simulink library "xps_library"  (R2021a)
settings: Solver=VariableStepAuto  StartTime=0.0  StopTime=10.0  RelTol=1e-3
undefined symbols (not defined in the file): ip_name, lib_path
libraries: xbsIndex_r4 x2612, casper_library_flow_control x68, simulink x52, $bdroot x9, casper_library_misc x9
(part 6 of 33)

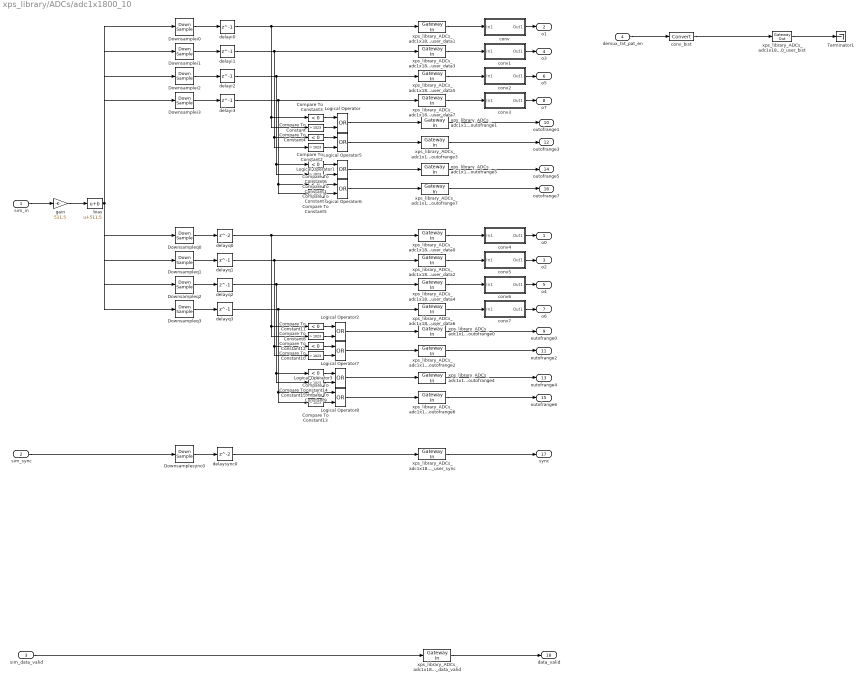
== system xps_library/ADCs/adc1x1800_10 ==
  sim_in : Inport  SampleTime=sample_period/8
  sim_sync : Inport  Port=2  SampleTime=sample_period/8
  sim_data_valid : Inport  Port=3  SampleTime=sample_period/4
  demux_tst_pat_en : Inport  Port=4  SampleTime=sample_period/8
  Compare To Constant{,1..2,5,8..10,13} (8 alike) : simulink/Logic and Bit Operations/Compare To Constant  relop=>  const=1023  OutDataTypeStr=boolean  ZeroCross=off
  Compare To Constant{3..4,6..7,11..12,14..15} (8 alike) : simulink/Logic and Bit Operations/Compare To Constant  relop=<  const=0  OutDataTypeStr=boolean  ZeroCross=off
  Downsamplei0 : DownSample  N=8  phase=1  InputProcessing=Inherited (this choice will be removed - see release notes)
  Downsamplei1 : DownSample  N=8  phase=3  InputProcessing=Inherited (this choice will be removed - see release notes)
  Downsamplei2 : DownSample  N=8  phase=5  InputProcessing=Inherited (this choice will be removed - see release notes)
  Downsamplei3 : DownSample  N=8  phase=7  InputProcessing=Inherited (this choice will be removed - see release notes)
  Downsampleq0 : DownSample  N=8  InputProcessing=Inherited (this choice will be removed - see release notes)
  Downsampleq1 : DownSample  N=8  phase=2  InputProcessing=Inherited (this choice will be removed - see release notes)
  Downsampleq2 : DownSample  N=8  phase=4  InputProcessing=Inherited (this choice will be removed - see release notes)
  Downsampleq3 : DownSample  N=8  phase=6  InputProcessing=Inherited (this choice will be removed - see release notes)
  Downsamplesync0 : DownSample  N=8  InputProcessing=Inherited (this choice will be removed - see release notes)
  Logical Operator{,1..3,5..8} (8 alike) : Logic  Operator=OR  AllPortsSameDT=off  OutDataTypeStr=boolean
  Terminator1 : Terminator
  bias : Bias  Bias=511.5  SaturateOnIntegerOverflow=on
  conv : Subsystem
  conv1 : Subsystem
  conv2 : Subsystem
  conv3 : Subsystem
  conv4 : Subsystem
  conv5 : Subsystem
  conv6 : Subsystem
  conv7 : Subsystem
  conv_bist : xbsIndex_r4/Convert  gui_display_data_type=Fixed-point  arith_type=Boolean  n_bits=8  bin_pt=0  float_type=Single  exp_bits=8  fraction_bits=24  quantization=Truncate  overflow=Wrap  en=off  latency=0  pipeline=off  dbl_ovrd=off  block_type=convert
      settings: xl_area=[0, 0, 0, 0, 0, 0, 0]
  delayi{0..3} (4 alike) : Delay  DelayLength=1
  delayq0 : Delay
  delayq1 : Delay  DelayLength=1
  delayq2 : Delay  DelayLength=1
  delayq3 : Delay  DelayLength=1
  delaysync0 : Delay
  gain : Gain  Gain=511.5  SaturateOnIntegerOverflow=on  OutDataTypeStr=Inherit: Same as input  ParamDataTypeStr=Inherit: Same as input
  xps_library_ADCs_adc1x1800_10_user_bist : xbsIndex_r4/Gateway Out  inherit_from_input=off  hdl_port=on  rows=1  columns=1  UseAsDAC=off  DACChannel='1'  interface=None  automatic_assignment=on  address_offset=hex2dec('00')  intf_name=''  intf_description=''  timing_constraint=None  locs_specified=off  LOCs={}  io_standard={}  block_type=gatewayout
      settings: infoedit="Gateway out block.  Converts Xilinx fixed point inputs into ouputs of type Simulink integer, double, or fixed point.<br><br>Hardware notes:  In hardware these blocks become top level output ports or are discarded, depending on how they are configured."  block_version=11.4
  xps_library_ADCs_adc1x1800_10_user_data{0..7} (8 alike) : xbsIndex_r4/Gateway In  gui_display_data_type=Fixed-point  arith_type=Unsigned  n_bits=10  bin_pt=0  preci_type=Single  exp_width=8  frac_width=24  rows=1  columns=1  quantization="Round  (unbiased: +/- Inf)"  overflow=Saturate  period=sample_period  UseAsADC=off  ADCChannel='1'  interface=None  automatic_assignment=on  address_offset=hex2dec('00')  intf_name=''  intf_description=''  default_value=0  timing_constraint=None  locs_specified=off  LOCs={}  io_standard={}  inherit_from_input=off  hdl_port=on  dbl_ovrd=off  block_type=gatewayin
      settings: infoedit="Gateway in block.  Converts inputs of type Simulink integer, double and fixed point to  Xilinx fixed point type.<br><br>Hardware notes:  In hardware these blocks become top level input ports."  xl_area=[0 0 0 0 8 0 0]  block_version=8.2.02
  xps_library_ADCs_adc1x1800_10_user_data_valid : xbsIndex_r4/Gateway In  gui_display_data_type=Fixed-point  arith_type=Boolean  n_bits=8  bin_pt=0  preci_type=Single  exp_width=8  frac_width=24  rows=1  columns=1  quantization="Round  (unbiased: +/- Inf)"  overflow=Saturate  period=sample_period  UseAsADC=off  ADCChannel='1'  interface=None  automatic_assignment=on  address_offset=hex2dec('00')  intf_name=''  intf_description=''  default_value=0  timing_constraint=None  locs_specified=off  LOCs={}  io_standard={}  inherit_from_input=off  hdl_port=on  dbl_ovrd=off  block_type=gatewayin
      settings: infoedit="Gateway in block.  Converts inputs of type Simulink integer, double and fixed point to  Xilinx fixed point type.<P><P>Hardware notes:  In hardware these blocks become top level input ports."  xl_area=[0 0 0 0 8 0 0]  block_version=8.2.02
  xps_library_ADCs_adc1x1800_10_user_outofrange{0..7} (8 alike) : xbsIndex_r4/Gateway In  gui_display_data_type=Fixed-point  arith_type=Boolean  n_bits=8  bin_pt=0  preci_type=Single  exp_width=8  frac_width=24  rows=1  columns=1  quantization="Round  (unbiased: +/- Inf)"  overflow=Saturate  period=sample_period  UseAsADC=off  ADCChannel='1'  interface=None  automatic_assignment=on  address_offset=hex2dec('00')  intf_name=''  intf_description=''  default_value=0  timing_constraint=None  locs_specified=off  LOCs={}  io_standard={}  inherit_from_input=off  hdl_port=on  dbl_ovrd=off  block_type=gatewayin
      settings: infoedit="Gateway in block.  Converts inputs of type Simulink integer, double and fixed point to  Xilinx fixed point type.<P><P>Hardware notes:  In hardware these blocks become top level input ports."  xl_area=[0 0 0 0 8 0 0]  block_version=8.2.02
  xps_library_ADCs_adc1x1800_10_user_sync : xbsIndex_r4/Gateway In  gui_display_data_type=Fixed-point  arith_type=Boolean  n_bits=8  bin_pt=0  preci_type=Single  exp_width=8  frac_width=24  rows=1  columns=1  quantization="Round  (unbiased: +/- Inf)"  overflow=Saturate  period=sample_period  UseAsADC=off  ADCChannel='1'  interface=None  automatic_assignment=on  address_offset=hex2dec('00')  intf_name=''  intf_description=''  default_value=0  timing_constraint=None  locs_specified=off  LOCs={}  io_standard={}  inherit_from_input=off  hdl_port=on  dbl_ovrd=off  block_type=gatewayin
      settings: infoedit="Gateway in block.  Converts inputs of type Simulink integer, double and fixed point to  Xilinx fixed point type.<P><P>Hardware notes:  In hardware these blocks become top level input ports."  xl_area=[0 0 0 0 8 0 0]  block_version=8.2.02
  o0 : Outport
  o1 : Outport  Port=2
  o2 : Outport  Port=3
  o3 : Outport  Port=4
  o4 : Outport  Port=5
  o5 : Outport  Port=6
  o6 : Outport  Port=7
  o7 : Outport  Port=8
  outofrange0 : Outport  Port=9
  outofrange1 : Outport  Port=10
  outofrange2 : Outport  Port=11
  outofrange3 : Outport  Port=12
  outofrange4 : Outport  Port=13
  outofrange5 : Outport  Port=14
  outofrange6 : Outport  Port=15
  outofrange7 : Outport  Port=16
  sync : Outport  Port=17
  data_valid : Outport  Port=18
  wires:
  delayq3/1 -> xps_library_ADCs_adc1x1800_10_user_data6/1, Compare To Constant15/1, Compare To Constant13/1
  delayq2/1 -> xps_library_ADCs_adc1x1800_10_user_data4/1, Compare To Constant14/1, Compare To Constant9/1
  delayq1/1 -> xps_library_ADCs_adc1x1800_10_user_data2/1, Compare To Constant12/1, Compare To Constant10/1
  delayi3/1 -> xps_library_ADCs_adc1x1800_10_user_data7/1, Compare To Constant7/1, Compare To Constant5/1
  delayi2/1 -> xps_library_ADCs_adc1x1800_10_user_data5/1, Compare To Constant6/1, Compare To Constant1/1
  delayi1/1 -> xps_library_ADCs_adc1x1800_10_user_data3/1, Compare To Constant2/1, Compare To Constant4/1
  Downsamplei0/1 -> delayi0/1
  xps_library_ADCs_adc1x1800_10_user_data6/1 -> conv7/1(In1)
  xps_library_ADCs_adc1x1800_10_user_data4/1 -> conv6/1(In1)
  xps_library_ADCs_adc1x1800_10_user_data2/1 -> conv5/1(In1)
  xps_library_ADCs_adc1x1800_10_user_data0/1 -> conv4/1(In1)
  xps_library_ADCs_adc1x1800_10_user_sync/1 -> sync/1
  xps_library_ADCs_adc1x1800_10_user_outofrange1/1 -> outofrange1/1
  xps_library_ADCs_adc1x1800_10_user_data7/1 -> conv3/1(In1)
  xps_library_ADCs_adc1x1800_10_user_data5/1 -> conv2/1(In1)
  xps_library_ADCs_adc1x1800_10_user_data3/1 -> conv1/1(In1)
  Downsampleq3/1 -> delayq3/1
  Downsampleq2/1 -> delayq2/1
  Downsampleq1/1 -> delayq1/1
  Downsamplei3/1 -> delayi3/1
  Downsamplei2/1 -> delayi2/1
  Downsamplei1/1 -> delayi1/1
  delayi0/1 -> xps_library_ADCs_adc1x1800_10_user_data1/1, Compare To Constant/1, Compare To Constant3/1
  Downsampleq0/1 -> delayq0/1
  delayq0/1 -> xps_library_ADCs_adc1x1800_10_user_data0/1, Compare To Constant11/1, Compare To Constant8/1
  Compare To Constant3/1 -> Logical Operator/1
  Compare To Constant/1 -> Logical Operator/2
  Compare To Constant4/1 -> Logical Operator5/1
  Compare To Constant2/1 -> Logical Operator5/2
  Logical Operator/1 -> xps_library_ADCs_adc1x1800_10_user_outofrange1/1
  Compare To Constant6/1 -> Logical Operator1/1
  Compare To Constant1/1 -> Logical Operator1/2
  Compare To Constant7/1 -> Logical Operator6/1
  Compare To Constant5/1 -> Logical Operator6/2
  Compare To Constant11/1 -> Logical Operator2/1
  Compare To Constant8/1 -> Logical Operator2/2
  Compare To Constant12/1 -> Logical Operator7/1
  Compare To Constant10/1 -> Logical Operator7/2
  Compare To Constant14/1 -> Logical Operator3/1
  Compare To Constant9/1 -> Logical Operator3/2
  Compare To Constant15/1 -> Logical Operator8/1
  Compare To Constant13/1 -> Logical Operator8/2
  sim_sync/1 -> Downsamplesync0/1
  Downsamplesync0/1 -> delaysync0/1
  delaysync0/1 -> xps_library_ADCs_adc1x1800_10_user_sync/1
  xps_library_ADCs_adc1x1800_10_user_data1/1 -> conv/1(In1)
  sim_in/1 -> gain/1
  gain/1 -> bias/1
  bias/1 -> Downsamplei0/1, Downsamplei1/1, Downsamplei2/1, Downsamplei3/1, Downsampleq0/1, Downsampleq1/1, Downsampleq2/1, Downsampleq3/1
  xps_library_ADCs_adc1x1800_10_user_outofrange3/1 -> outofrange3/1
  Logical Operator5/1 -> xps_library_ADCs_adc1x1800_10_user_outofrange3/1
  xps_library_ADCs_adc1x1800_10_user_outofrange5/1 -> outofrange5/1
  Logical Operator1/1 -> xps_library_ADCs_adc1x1800_10_user_outofrange5/1
  xps_library_ADCs_adc1x1800_10_user_outofrange7/1 -> outofrange7/1
  Logical Operator6/1 -> xps_library_ADCs_adc1x1800_10_user_outofrange7/1
  xps_library_ADCs_adc1x1800_10_user_outofrange0/1 -> outofrange0/1
  Logical Operator2/1 -> xps_library_ADCs_adc1x1800_10_user_outofrange0/1
  xps_library_ADCs_adc1x1800_10_user_outofrange2/1 -> outofrange2/1
  Logical Operator7/1 -> xps_library_ADCs_adc1x1800_10_user_outofrange2/1
  xps_library_ADCs_adc1x1800_10_user_outofrange4/1 -> outofrange4/1
  Logical Operator3/1 -> xps_library_ADCs_adc1x1800_10_user_outofrange4/1
  xps_library_ADCs_adc1x1800_10_user_outofrange6/1 -> outofrange6/1
  Logical Operator8/1 -> xps_library_ADCs_adc1x1800_10_user_outofrange6/1
  xps_library_ADCs_adc1x1800_10_user_data_valid/1 -> data_valid/1
  sim_data_valid/1 -> xps_library_ADCs_adc1x1800_10_user_data_valid/1
  demux_tst_pat_en/1 -> conv_bist/1
  xps_library_ADCs_adc1x1800_10_user_bist/1 -> Terminator1/1
  conv_bist/1 -> xps_library_ADCs_adc1x1800_10_user_bist/1
  conv/1(Out1) -> o1/1
  conv1/1(Out1) -> o3/1
  conv2/1(Out1) -> o5/1
  conv3/1(Out1) -> o7/1
  conv4/1(Out1) -> o0/1
  conv5/1(Out1) -> o2/1
  conv6/1(Out1) -> o4/1
  conv7/1(Out1) -> o6/1

== system xps_library/ADCs/adc2x14_400 ==
  conv : Subsystem
      mask help:
      | Converts an (12-bit) unsigned number to 2's complement.
      | This block should eventually be able to handle arbitrary
      | width inputs.
  conv1 : Subsystem
      mask help:
      | Converts an (12-bit) unsigned number to 2's complement.
      | This block should eventually be able to handle arbitrary
      | width inputs.
  conv2 : Subsystem
      mask help:
      | Converts an (12-bit) unsigned number to 2's complement.
      | This block should eventually be able to handle arbitrary
      | width inputs.
  conv3 : Subsystem
      mask help:
      | Converts an (12-bit) unsigned number to 2's complement.
      | This block should eventually be able to handle arbitrary
      | width inputs.
  xps_library_ADCs_adc2x14_400_user_data_i0 : xbsIndex_r4/Gateway In  gui_display_data_type=Fixed-point  arith_type=Unsigned  n_bits=14  bin_pt=0  preci_type=Single  exp_width=8  frac_width=24  rows=1  columns=1  quantization=Truncate  overflow=Wrap  period=1  UseAsADC=off  ADCChannel='1'  interface=None  automatic_assignment=on  address_offset=hex2dec('00')  intf_name=''  intf_description=''  default_value=0  timing_constraint=None  locs_specified=off  LOCs={}  io_standard={}  inherit_from_input=off  hdl_port=on  dbl_ovrd=off  block_type=gatewayin
      settings: infoedit="Gateway in block.  Converts inputs of type Simulink integer, double and fixed point to  Xilinx fixed point type.<P><P>Hardware notes:  In hardware these blocks become top level input ports."  xl_area=[0, 0, 0, 0, 0, 0, 0]  block_version=10.1.3
  xps_library_ADCs_adc2x14_400_user_data_i1 : xbsIndex_r4/Gateway In  gui_display_data_type=Fixed-point  arith_type=Unsigned  n_bits=14  bin_pt=0  preci_type=Single  exp_width=8  frac_width=24  rows=1  columns=1  quantization=Truncate  overflow=Wrap  period=1  UseAsADC=off  ADCChannel='1'  interface=None  automatic_assignment=on  address_offset=hex2dec('00')  intf_name=''  intf_description=''  default_value=0  timing_constraint=None  locs_specified=off  LOCs={}  io_standard={}  inherit_from_input=off  hdl_port=on  dbl_ovrd=off  block_type=gatewayin
      settings: infoedit="Gateway in block.  Converts inputs of type Simulink integer, double and fixed point to  Xilinx fixed point type.<P><P>Hardware notes:  In hardware these blocks become top level input ports."  xl_area=[0, 0, 0, 0, 0, 0, 0]  block_version=10.1.3
  xps_library_ADCs_adc2x14_400_user_data_q0 : xbsIndex_r4/Gateway In  gui_display_data_type=Fixed-point  arith_type=Unsigned  n_bits=14  bin_pt=0  preci_type=Single  exp_width=8  frac_width=24  rows=1  columns=1  quantization=Truncate  overflow=Wrap  period=1  UseAsADC=off  ADCChannel='1'  interface=None  automatic_assignment=on  address_offset=hex2dec('00')  intf_name=''  intf_description=''  default_value=0  timing_constraint=None  locs_specified=off  LOCs={}  io_standard={}  inherit_from_input=off  hdl_port=on  dbl_ovrd=off  block_type=gatewayin
      settings: infoedit="Gateway in block.  Converts inputs of type Simulink integer, double and fixed point to  Xilinx fixed point type.<P><P>Hardware notes:  In hardware these blocks become top level input ports."  xl_area=[0, 0, 0, 0, 0, 0, 0]  block_version=10.1.3
  xps_library_ADCs_adc2x14_400_user_data_q1 : xbsIndex_r4/Gateway In  gui_display_data_type=Fixed-point  arith_type=Unsigned  n_bits=14  bin_pt=0  preci_type=Single  exp_width=8  frac_width=24  rows=1  columns=1  quantization=Truncate  overflow=Wrap  period=1  UseAsADC=off  ADCChannel='1'  interface=None  automatic_assignment=on  address_offset=hex2dec('00')  intf_name=''  intf_description=''  default_value=0  timing_constraint=None  locs_specified=off  LOCs={}  io_standard={}  inherit_from_input=off  hdl_port=on  dbl_ovrd=off  block_type=gatewayin
      settings: infoedit="Gateway in block.  Converts inputs of type Simulink integer, double and fixed point to  Xilinx fixed point type.<P><P>Hardware notes:  In hardware these blocks become top level input ports."  xl_area=[0, 0, 0, 0, 0, 0, 0]  block_version=10.1.3
  xps_library_ADCs_adc2x14_400_user_sync : xbsIndex_r4/Gateway In  gui_display_data_type=Fixed-point  arith_type=Boolean  n_bits=1  bin_pt=0  preci_type=Single  exp_width=8  frac_width=24  rows=1  columns=1  quantization=Truncate  overflow=Wrap  period=1  UseAsADC=off  ADCChannel='1'  interface=None  automatic_assignment=on  address_offset=hex2dec('00')  intf_name=''  intf_description=''  default_value=0  timing_constraint=None  locs_specified=off  LOCs={}  io_standard={}  inherit_from_input=off  hdl_port=on  dbl_ovrd=off  block_type=gatewayin
      settings: infoedit="Gateway in block.  Converts inputs of type Simulink integer, double and fixed point to  Xilinx fixed point type.<P><P>Hardware notes:  In hardware these blocks become top level input ports."  xl_area=[0, 0, 0, 0, 0, 0, 0]  block_version=10.1.3
  data_i0 : Outport
  data_i1 : Outport  Port=2
  data_q0 : Outport  Port=3
  data_q1 : Outport  Port=4
  sync : Outport  Port=5
  wires:
  xps_library_ADCs_adc2x14_400_user_sync/1 -> sync/1
  xps_library_ADCs_adc2x14_400_user_data_i0/1 -> conv/1(In1)
  conv/1(Out1) -> data_i0/1
  xps_library_ADCs_adc2x14_400_user_data_q0/1 -> conv2/1(In1)
  conv2/1(Out1) -> data_q0/1
  xps_library_ADCs_adc2x14_400_user_data_i1/1 -> conv1/1(In1)
  conv1/1(Out1) -> data_i1/1
  xps_library_ADCs_adc2x14_400_user_data_q1/1 -> conv3/1(In1)
  conv3/1(Out1) -> data_q1/1

== system xps_library/ADCs/adc2x14_400_4x ==
  conv : Subsystem
      mask help:
      | Converts an (14-bit) unsigned number to 2's complement.
      | This block should eventually be able to handle arbitrary
      | width inputs.
  conv1 : Subsystem
      mask help:
      | Converts an (14-bit) unsigned number to 2's complement.
      | This block should eventually be able to handle arbitrary
      | width inputs.
  conv2 : Subsystem
      mask help:
      | Converts an (14-bit) unsigned number to 2's complement.
      | This block should eventually be able to handle arbitrary
      | width inputs.
  conv3 : Subsystem
      mask help:
      | Converts an (14-bit) unsigned number to 2's complement.
      | This block should eventually be able to handle arbitrary
      | width inputs.
  conv4 : Subsystem
      mask help:
      | Converts an (14-bit) unsigned number to 2's complement.
      | This block should eventually be able to handle arbitrary
      | width inputs.
  conv5 : Subsystem
      mask help:
      | Converts an (14-bit) unsigned number to 2's complement.
      | This block should eventually be able to handle arbitrary
      | width inputs.
  conv6 : Subsystem
      mask help:
      | Converts an (14-bit) unsigned number to 2's complement.
      | This block should eventually be able to handle arbitrary
      | width inputs.
  conv7 : Subsystem
      mask help:
      | Converts an (14-bit) unsigned number to 2's complement.
      | This block should eventually be able to handle arbitrary
      | width inputs.
  xps_library_ADCs_adc2x14_400_4x_user_data_i{0..3} (4 alike) : xbsIndex_r4/Gateway In  gui_display_data_type=Fixed-point  arith_type=Unsigned  n_bits=14  bin_pt=0  preci_type=Single  exp_width=8  frac_width=24  rows=1  columns=1  quantization=Truncate  overflow=Wrap  period=1  UseAsADC=off  ADCChannel='1'  interface=None  automatic_assignment=on  address_offset=hex2dec('00')  intf_name=''  intf_description=''  default_value=0  timing_constraint=None  locs_specified=off  LOCs={}  io_standard={}  inherit_from_input=off  hdl_port=on  dbl_ovrd=off  block_type=gatewayin
      settings: infoedit="Gateway in block.  Converts inputs of type Simulink integer, double and fixed point to  Xilinx fixed point type.<P><P>Hardware notes:  In hardware these blocks become top level input ports."  xl_area=[0, 0, 0, 0, 0, 0, 0]  block_version=10.1.3
  xps_library_ADCs_adc2x14_400_4x_user_data_q{0..3} (4 alike) : xbsIndex_r4/Gateway In  gui_display_data_type=Fixed-point  arith_type=Unsigned  n_bits=14  bin_pt=0  preci_type=Single  exp_width=8  frac_width=24  rows=1  columns=1  quantization=Truncate  overflow=Wrap  period=1  UseAsADC=off  ADCChannel='1'  interface=None  automatic_assignment=on  address_offset=hex2dec('00')  intf_name=''  intf_description=''  default_value=0  timing_constraint=None  locs_specified=off  LOCs={}  io_standard={}  inherit_from_input=off  hdl_port=on  dbl_ovrd=off  block_type=gatewayin
      settings: infoedit="Gateway in block.  Converts inputs of type Simulink integer, double and fixed point to  Xilinx fixed point type.<P><P>Hardware notes:  In hardware these blocks become top level input ports."  xl_area=[0, 0, 0, 0, 0, 0, 0]  block_version=10.1.3
  xps_library_ADCs_adc2x14_400_4x_user_sync : xbsIndex_r4/Gateway In  gui_display_data_type=Fixed-point  arith_type=Boolean  n_bits=1  bin_pt=0  preci_type=Single  exp_width=8  frac_width=24  rows=1  columns=1  quantization=Truncate  overflow=Wrap  period=1  UseAsADC=off  ADCChannel='1'  interface=None  automatic_assignment=on  address_offset=hex2dec('00')  intf_name=''  intf_description=''  default_value=0  timing_constraint=None  locs_specified=off  LOCs={}  io_standard={}  inherit_from_input=off  hdl_port=on  dbl_ovrd=off  block_type=gatewayin
      settings: infoedit="Gateway in block.  Converts inputs of type Simulink integer, double and fixed point to  Xilinx fixed point type.<P><P>Hardware notes:  In hardware these blocks become top level input ports."  xl_area=[0, 0, 0, 0, 0, 0, 0]  block_version=10.1.3
  data_i0 : Outport
  data_i1 : Outport  Port=2
  data_i2 : Outport  Port=3
  data_i3 : Outport  Port=4
  data_q0 : Outport  Port=5
  data_q1 : Outport  Port=6
  data_q2 : Outport  Port=7
  data_q3 : Outport  Port=8
  sync : Outport  Port=9
  wires:
  conv5/1(Out1) -> data_q1/1
  xps_library_ADCs_adc2x14_400_4x_user_data_q1/1 -> conv5/1(In1)
  conv1/1(Out1) -> data_i1/1
  xps_library_ADCs_adc2x14_400_4x_user_data_i1/1 -> conv1/1(In1)
  conv4/1(Out1) -> data_q0/1
  xps_library_ADCs_adc2x14_400_4x_user_data_q0/1 -> conv4/1(In1)
  conv/1(Out1) -> data_i0/1
  xps_library_ADCs_adc2x14_400_4x_user_data_i0/1 -> conv/1(In1)
  xps_library_ADCs_adc2x14_400_4x_user_sync/1 -> sync/1
  conv2/1(Out1) -> data_i2/1
  xps_library_ADCs_adc2x14_400_4x_user_data_i2/1 -> conv2/1(In1)
  conv3/1(Out1) -> data_i3/1
  xps_library_ADCs_adc2x14_400_4x_user_data_i3/1 -> conv3/1(In1)
  conv6/1(Out1) -> data_q2/1
  xps_library_ADCs_adc2x14_400_4x_user_data_q2/1 -> conv6/1(In1)
  conv7/1(Out1) -> data_q3/1
  xps_library_ADCs_adc2x14_400_4x_user_data_q3/1 -> conv7/1(In1)

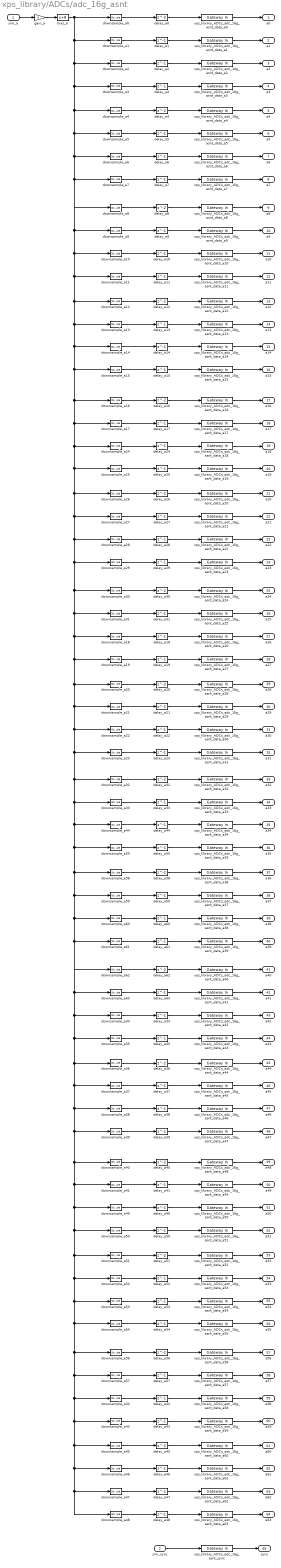
== system xps_library/ADCs/adc_16g_asnt ==
  sim_a : Inport
  sim_sync : Inport  Port=2
  bias_a : Bias  Bias=8  SaturateOnIntegerOverflow=on
  delay_a{0,4,8,12,16,20,26,30,32,36,40,45,51,56,58,62} (16 alike) : Delay  InitialCondition=0
  delay_a{1..3,5..7,9..11,13..15,17..19,21..25,27..29,31,33..35,37..39,41..44,46..50,52..55,57,59..61,63} (48 alike) : Delay  DelayLength=1  InitialCondition=0
  downsample_a{0,4,8,12,16,20,26,30,32,36,40,45,51,56,58,62} (16 alike) : DownSample  N=64  RateOptions=Allow multirate processing
  downsample_a{1,5,9,13,17,21,27,31,33,37,41,46,52,57,59,63} (16 alike) : DownSample  N=64  phase=1  RateOptions=Allow multirate processing
  downsample_a{2,6,10,14,18,22,24,28,34,38,42,44,47,49,53,60} (16 alike) : DownSample  N=64  phase=2  RateOptions=Allow multirate processing
  downsample_a{3,7,11,15,19,23,25,29,35,39,43,48,50,54..55,61} (16 alike) : DownSample  N=64  phase=3  RateOptions=Allow multirate processing
  gain_a : Gain  Gain=8  SaturateOnIntegerOverflow=on  OutDataTypeStr=Inherit: Same as input  ParamDataTypeStr=Inherit: Same as input
  xps_library_ADCs_adc_16g_asnt_data_a{0..63} (64 alike) : xbsIndex_r4/Gateway In  gui_display_data_type=Fixed-point  arith_type=Unsigned  n_bits=4  bin_pt=0  preci_type=Single  exp_width=8  frac_width=24  rows=1  columns=1  quantization=Truncate  overflow=Wrap  period=1  UseAsADC=off  ADCChannel='1'  interface=None  automatic_assignment=on  address_offset=hex2dec('00')  intf_name=''  intf_description=''  default_value=0  timing_constraint=None  locs_specified=off  LOCs={}  io_standard={}  inherit_from_input=off  hdl_port=on  dbl_ovrd=off  block_type=gatewayin
  xps_library_ADCs_adc_16g_asnt_sync : xbsIndex_r4/Gateway In  gui_display_data_type=Fixed-point  arith_type=Boolean  n_bits=16  bin_pt=14  preci_type=Single  exp_width=8  frac_width=24  rows=1  columns=1  quantization="Round  (unbiased: +/- Inf)"  overflow=Saturate  period=1  UseAsADC=off  ADCChannel='1'  interface=None  automatic_assignment=on  address_offset=hex2dec('00')  intf_name=''  intf_description=''  default_value=0  timing_constraint=None  locs_specified=off  LOCs={}  io_standard={}  inherit_from_input=off  hdl_port=on  dbl_ovrd=off  block_type=gatewayin
  a0 : Outport  VectorParamsAs1DForOutWhenUnconnected=off
  a1 : Outport  Port=2  VectorParamsAs1DForOutWhenUnconnected=off
  a2 : Outport  Port=3  VectorParamsAs1DForOutWhenUnconnected=off
  a3 : Outport  Port=4  VectorParamsAs1DForOutWhenUnconnected=off
  a4 : Outport  Port=5  VectorParamsAs1DForOutWhenUnconnected=off
  a5 : Outport  Port=6  VectorParamsAs1DForOutWhenUnconnected=off
  a6 : Outport  Port=7  VectorParamsAs1DForOutWhenUnconnected=off
  a7 : Outport  Port=8  VectorParamsAs1DForOutWhenUnconnected=off
  a8 : Outport  Port=9  VectorParamsAs1DForOutWhenUnconnected=off
  a9 : Outport  Port=10  VectorParamsAs1DForOutWhenUnconnected=off
  a10 : Outport  Port=11  VectorParamsAs1DForOutWhenUnconnected=off
  a11 : Outport  Port=12  VectorParamsAs1DForOutWhenUnconnected=off
  a12 : Outport  Port=13  VectorParamsAs1DForOutWhenUnconnected=off
  a13 : Outport  Port=14  VectorParamsAs1DForOutWhenUnconnected=off
  a14 : Outport  Port=15  VectorParamsAs1DForOutWhenUnconnected=off
  a15 : Outport  Port=16  VectorParamsAs1DForOutWhenUnconnected=off
  a16 : Outport  Port=17  VectorParamsAs1DForOutWhenUnconnected=off
  a17 : Outport  Port=18  VectorParamsAs1DForOutWhenUnconnected=off
  a18 : Outport  Port=19  VectorParamsAs1DForOutWhenUnconnected=off
  a19 : Outport  Port=20  VectorParamsAs1DForOutWhenUnconnected=off
  a20 : Outport  Port=21  VectorParamsAs1DForOutWhenUnconnected=off
  a21 : Outport  Port=22  VectorParamsAs1DForOutWhenUnconnected=off
  a22 : Outport  Port=23  VectorParamsAs1DForOutWhenUnconnected=off
  a23 : Outport  Port=24  VectorParamsAs1DForOutWhenUnconnected=off
  a24 : Outport  Port=25  VectorParamsAs1DForOutWhenUnconnected=off
  a25 : Outport  Port=26  VectorParamsAs1DForOutWhenUnconnected=off
  a26 : Outport  Port=27  VectorParamsAs1DForOutWhenUnconnected=off
  a27 : Outport  Port=28  VectorParamsAs1DForOutWhenUnconnected=off
  a28 : Outport  Port=29  VectorParamsAs1DForOutWhenUnconnected=off
  a29 : Outport  Port=30  VectorParamsAs1DForOutWhenUnconnected=off
  a30 : Outport  Port=31  VectorParamsAs1DForOutWhenUnconnected=off
  a31 : Outport  Port=32  VectorParamsAs1DForOutWhenUnconnected=off
  a32 : Outport  Port=33  VectorParamsAs1DForOutWhenUnconnected=off
  a33 : Outport  Port=34  VectorParamsAs1DForOutWhenUnconnected=off
  a34 : Outport  Port=35  VectorParamsAs1DForOutWhenUnconnected=off
  a35 : Outport  Port=36  VectorParamsAs1DForOutWhenUnconnected=off
  a36 : Outport  Port=37  VectorParamsAs1DForOutWhenUnconnected=off
  a37 : Outport  Port=38  VectorParamsAs1DForOutWhenUnconnected=off
  a38 : Outport  Port=39  VectorParamsAs1DForOutWhenUnconnected=off
  a39 : Outport  Port=40  VectorParamsAs1DForOutWhenUnconnected=off
  a40 : Outport  Port=41  VectorParamsAs1DForOutWhenUnconnected=off
  a41 : Outport  Port=42  VectorParamsAs1DForOutWhenUnconnected=off
  a42 : Outport  Port=43  VectorParamsAs1DForOutWhenUnconnected=off
  a43 : Outport  Port=44  VectorParamsAs1DForOutWhenUnconnected=off
  a44 : Outport  Port=45  VectorParamsAs1DForOutWhenUnconnected=off
  a45 : Outport  Port=46  VectorParamsAs1DForOutWhenUnconnected=off
  a46 : Outport  Port=47  VectorParamsAs1DForOutWhenUnconnected=off
  a47 : Outport  Port=48  VectorParamsAs1DForOutWhenUnconnected=off
  a48 : Outport  Port=49  VectorParamsAs1DForOutWhenUnconnected=off
  a49 : Outport  Port=50  VectorParamsAs1DForOutWhenUnconnected=off
  a50 : Outport  Port=51  VectorParamsAs1DForOutWhenUnconnected=off
  a51 : Outport  Port=52  VectorParamsAs1DForOutWhenUnconnected=off
  a52 : Outport  Port=53  VectorParamsAs1DForOutWhenUnconnected=off
  a53 : Outport  Port=54  VectorParamsAs1DForOutWhenUnconnected=off
  a54 : Outport  Port=55  VectorParamsAs1DForOutWhenUnconnected=off
  a55 : Outport  Port=56  VectorParamsAs1DForOutWhenUnconnected=off
  a56 : Outport  Port=57  VectorParamsAs1DForOutWhenUnconnected=off
  a57 : Outport  Port=58  VectorParamsAs1DForOutWhenUnconnected=off
  a58 : Outport  Port=59  VectorParamsAs1DForOutWhenUnconnected=off
  a59 : Outport  Port=60  VectorParamsAs1DForOutWhenUnconnected=off
  a60 : Outport  Port=61  VectorParamsAs1DForOutWhenUnconnected=off
  a61 : Outport  Port=62  VectorParamsAs1DForOutWhenUnconnected=off
  a62 : Outport  Port=63  VectorParamsAs1DForOutWhenUnconnected=off
  a63 : Outport  Port=64  VectorParamsAs1DForOutWhenUnconnected=off
  sync : Outport  Port=65  VectorParamsAs1DForOutWhenUnconnected=off
  wires:
  xps_library_ADCs_adc_16g_asnt_sync/1 -> sync/1
  delay_a58/1 -> xps_library_ADCs_adc_16g_asnt_data_a36/1
  xps_library_ADCs_adc_16g_asnt_data_a46/1 -> a46/1
  delay_a54/1 -> xps_library_ADCs_adc_16g_asnt_data_a55/1
  delay_a44/1 -> xps_library_ADCs_adc_16g_asnt_data_a34/1
  xps_library_ADCs_adc_16g_asnt_data_a34/1 -> a34/1
  delay_a55/1 -> xps_library_ADCs_adc_16g_asnt_data_a35/1
  downsample_a48/1 -> delay_a48/1
  bias_a/1 -> downsample_a7/1, downsample_a8/1, downsample_a6/1, downsample_a5/1, downsample_a4/1, downsample_a3/1, downsample_a1/1, downsample_a0/1, downsample_a2/1, downsample_a9/1, downsample_a10/1, downsample_a11/1, downsample_a12/1, downsample_a13/1, downsample_a14/1, downsample_a15/1, downsample_a16/1, downsample_a17/1, downsample_a24/1, downsample_a25/1, downsample_a26/1, downsample_a27/1, downsample_a28/1, downsample_a29/1, downsample_a30/1, downsample_a31/1, downsample_a18/1, downsample_a19/1, downsample_a20/1, downsample_a21/1, downsample_a22/1, downsample_a23/1, downsample_a61/1, downsample_a62/1, downsample_a60/1, downsample_a59/1, downsample_a58/1, downsample_a55/1, downsample_a33/1, downsample_a32/1, downsample_a63/1, downsample_a34/1, downsample_a35/1, downsample_a36/1, downsample_a37/1, downsample_a38/1, downsample_a39/1, downsample_a40/1, downsample_a41/1, downsample_a49/1, downsample_a50/1, downsample_a51/1, downsample_a52/1, downsample_a53/1, downsample_a54/1, downsample_a56/1, downsample_a57/1, downsample_a42/1, downsample_a43/1, downsample_a45/1, downsample_a48/1, downsample_a47/1, downsample_a46/1, downsample_a44/1
  xps_library_ADCs_adc_16g_asnt_data_a35/1 -> a35/1
  downsample_a33/1 -> delay_a33/1
  xps_library_ADCs_adc_16g_asnt_data_a32/1 -> a32/1
  delay_a33/1 -> xps_library_ADCs_adc_16g_asnt_data_a33/1
  xps_library_ADCs_adc_16g_asnt_data_a33/1 -> a33/1
  downsample_a44/1 -> delay_a44/1
  downsample_a55/1 -> delay_a55/1
  delay_a51/1 -> xps_library_ADCs_adc_16g_asnt_data_a52/1
  delay_a57/1 -> xps_library_ADCs_adc_16g_asnt_data_a57/1
  delay_a49/1 -> xps_library_ADCs_adc_16g_asnt_data_a50/1
  delay_a43/1 -> xps_library_ADCs_adc_16g_asnt_data_a59/1
  xps_library_ADCs_adc_16g_asnt_data_a54/1 -> a54/1
  downsample_a57/1 -> delay_a57/1
  delay_a52/1 -> xps_library_ADCs_adc_16g_asnt_data_a53/1
  downsample_a53/1 -> delay_a53/1
  xps_library_ADCs_adc_16g_asnt_data_a49/1 -> a49/1
  xps_library_ADCs_adc_16g_asnt_data_a51/1 -> a51/1
  delay_a32/1 -> xps_library_ADCs_adc_16g_asnt_data_a32/1
  downsample_a47/1 -> delay_a47/1
  xps_library_ADCs_adc_16g_asnt_data_a50/1 -> a50/1
  downsample_a41/1 -> delay_a41/1
  xps_library_ADCs_adc_16g_asnt_data_a45/1 -> a45/1
  xps_library_ADCs_adc_16g_asnt_data_a41/1 -> a41/1
  delay_a48/1 -> xps_library_ADCs_adc_16g_asnt_data_a63/1
  delay_a40/1 -> xps_library_ADCs_adc_16g_asnt_data_a48/1
  xps_library_ADCs_adc_16g_asnt_data_a59/1 -> a59/1
  downsample_a36/1 -> delay_a36/1
  xps_library_ADCs_adc_16g_asnt_data_a44/1 -> a44/1
  downsample_a38/1 -> delay_a38/1
  downsample_a34/1 -> delay_a34/1
  downsample_a32/1 -> delay_a32/1
  downsample_a39/1 -> delay_a39/1
  xps_library_ADCs_adc_16g_asnt_data_a57/1 -> a57/1
  delay_a36/1 -> xps_library_ADCs_adc_16g_asnt_data_a44/1
  delay_a35/1 -> xps_library_ADCs_adc_16g_asnt_data_a43/1
  delay_a45/1 -> xps_library_ADCs_adc_16g_asnt_data_a60/1
  xps_library_ADCs_adc_16g_asnt_data_a48/1 -> a48/1
  xps_library_ADCs_adc_16g_asnt_data_a58/1 -> a58/1
  delay_a59/1 -> xps_library_ADCs_adc_16g_asnt_data_a37/1
  delay_a46/1 -> xps_library_ADCs_adc_16g_asnt_data_a61/1
  delay_a60/1 -> xps_library_ADCs_adc_16g_asnt_data_a38/1
  xps_library_ADCs_adc_16g_asnt_data_a52/1 -> a52/1
  xps_library_ADCs_adc_16g_asnt_data_a39/1 -> a39/1
  delay_a41/1 -> xps_library_ADCs_adc_16g_asnt_data_a49/1
  downsample_a62/1 -> delay_a62/1
  xps_library_ADCs_adc_16g_asnt_data_a55/1 -> a55/1
  xps_library_ADCs_adc_16g_asnt_data_a63/1 -> a63/1
  xps_library_ADCs_adc_16g_asnt_data_a53/1 -> a53/1
  xps_library_ADCs_adc_16g_asnt_data_a61/1 -> a61/1
  xps_library_ADCs_adc_16g_asnt_data_a40/1 -> a40/1
  downsample_a40/1 -> delay_a40/1
  downsample_a51/1 -> delay_a51/1
  xps_library_ADCs_adc_16g_asnt_data_a43/1 -> a43/1
  delay_a47/1 -> xps_library_ADCs_adc_16g_asnt_data_a62/1
  delay_a63/1 -> xps_library_ADCs_adc_16g_asnt_data_a41/1
  downsample_a60/1 -> delay_a60/1
  delay_a56/1 -> xps_library_ADCs_adc_16g_asnt_data_a56/1
  xps_library_ADCs_adc_16g_asnt_data_a37/1 -> a37/1
  xps_library_ADCs_adc_16g_asnt_data_a60/1 -> a60/1
  delay_a61/1 -> xps_library_ADCs_adc_16g_asnt_data_a39/1
  delay_a62/1 -> xps_library_ADCs_adc_16g_asnt_data_a40/1
  downsample_a54/1 -> delay_a54/1
  downsample_a56/1 -> delay_a56/1
  xps_library_ADCs_adc_16g_asnt_data_a62/1 -> a62/1
  downsample_a35/1 -> delay_a35/1
  downsample_a58/1 -> delay_a58/1
  downsample_a52/1 -> delay_a52/1
  downsample_a45/1 -> delay_a45/1
  delay_a38/1 -> xps_library_ADCs_adc_16g_asnt_data_a46/1
  downsample_a42/1 -> delay_a42/1
  downsample_a43/1 -> delay_a43/1
  delay_a50/1 -> xps_library_ADCs_adc_16g_asnt_data_a51/1
  downsample_a63/1 -> delay_a63/1
  delay_a34/1 -> xps_library_ADCs_adc_16g_asnt_data_a42/1
  xps_library_ADCs_adc_16g_asnt_data_a47/1 -> a47/1
  delay_a37/1 -> xps_library_ADCs_adc_16g_asnt_data_a45/1
  downsample_a50/1 -> delay_a50/1
  xps_library_ADCs_adc_16g_asnt_data_a56/1 -> a56/1
  downsample_a49/1 -> delay_a49/1
  delay_a39/1 -> xps_library_ADCs_adc_16g_asnt_data_a47/1
  downsample_a37/1 -> delay_a37/1
  delay_a53/1 -> xps_library_ADCs_adc_16g_asnt_data_a54/1
  downsample_a46/1 -> delay_a46/1
  downsample_a61/1 -> delay_a61/1
  xps_library_ADCs_adc_16g_asnt_data_a42/1 -> a42/1
  xps_library_ADCs_adc_16g_asnt_data_a38/1 -> a38/1
  xps_library_ADCs_adc_16g_asnt_data_a36/1 -> a36/1
  delay_a42/1 -> xps_library_ADCs_adc_16g_asnt_data_a58/1
  downsample_a59/1 -> delay_a59/1
  delay_a26/1 -> xps_library_ADCs_adc_16g_asnt_data_a20/1
  xps_library_ADCs_adc_16g_asnt_data_a30/1 -> a30/1
  xps_library_ADCs_adc_16g_asnt_data_a28/1 -> a28/1
  downsample_a16/1 -> delay_a16/1
  delay_a24/1 -> xps_library_ADCs_adc_16g_asnt_data_a18/1
  delay_a16/1 -> xps_library_ADCs_adc_16g_asnt_data_a16/1
  xps_library_ADCs_adc_16g_asnt_data_a19/1 -> a19/1
  downsample_a17/1 -> delay_a17/1
  xps_library_ADCs_adc_16g_asnt_data_a16/1 -> a16/1
  delay_a17/1 -> xps_library_ADCs_adc_16g_asnt_data_a17/1
  xps_library_ADCs_adc_16g_asnt_data_a17/1 -> a17/1
  downsample_a24/1 -> delay_a24/1
  downsample_a25/1 -> delay_a25/1
  xps_library_ADCs_adc_16g_asnt_data_a23/1 -> a23/1
  delay_a29/1 -> xps_library_ADCs_adc_16g_asnt_data_a23/1
  delay_a19/1 -> xps_library_ADCs_adc_16g_asnt_data_a27/1
  xps_library_ADCs_adc_16g_asnt_data_a29/1 -> a29/1
  xps_library_ADCs_adc_16g_asnt_data_a26/1 -> a26/1
  downsample_a23/1 -> delay_a23/1
  downsample_a20/1 -> delay_a20/1
  delay_a20/1 -> xps_library_ADCs_adc_16g_asnt_data_a28/1
  xps_library_ADCs_adc_16g_asnt_data_a24/1 -> a24/1
  delay_a22/1 -> xps_library_ADCs_adc_16g_asnt_data_a30/1
  delay_a27/1 -> xps_library_ADCs_adc_16g_asnt_data_a21/1
  downsample_a31/1 -> delay_a31/1
  downsample_a28/1 -> delay_a28/1
  downsample_a30/1 -> delay_a30/1
  downsample_a18/1 -> delay_a18/1
  delay_a30/1 -> xps_library_ADCs_adc_16g_asnt_data_a24/1
  delay_a21/1 -> xps_library_ADCs_adc_16g_asnt_data_a29/1
  delay_a28/1 -> xps_library_ADCs_adc_16g_asnt_data_a22/1
  downsample_a26/1 -> delay_a26/1
  downsample_a22/1 -> delay_a22/1
  delay_a23/1 -> xps_library_ADCs_adc_16g_asnt_data_a31/1
  downsample_a19/1 -> delay_a19/1
  xps_library_ADCs_adc_16g_asnt_data_a18/1 -> a18/1
  xps_library_ADCs_adc_16g_asnt_data_a22/1 -> a22/1
  xps_library_ADCs_adc_16g_asnt_data_a25/1 -> a25/1
  downsample_a21/1 -> delay_a21/1
  delay_a18/1 -> xps_library_ADCs_adc_16g_asnt_data_a26/1
  xps_library_ADCs_adc_16g_asnt_data_a31/1 -> a31/1
  xps_library_ADCs_adc_16g_asnt_data_a20/1 -> a20/1
  downsample_a27/1 -> delay_a27/1
  downsample_a29/1 -> delay_a29/1
  xps_library_ADCs_adc_16g_asnt_data_a21/1 -> a21/1
  xps_library_ADCs_adc_16g_asnt_data_a27/1 -> a27/1
  delay_a31/1 -> xps_library_ADCs_adc_16g_asnt_data_a25/1
  delay_a25/1 -> xps_library_ADCs_adc_16g_asnt_data_a19/1
  downsample_a12/1 -> delay_a12/1
  delay_a14/1 -> xps_library_ADCs_adc_16g_asnt_data_a14/1
  delay_a15/1 -> xps_library_ADCs_adc_16g_asnt_data_a15/1
  delay_a13/1 -> xps_library_ADCs_adc_16g_asnt_data_a13/1
  downsample_a14/1 -> delay_a14/1
  xps_library_ADCs_adc_16g_asnt_data_a13/1 -> a13/1
  downsample_a15/1 -> delay_a15/1
  xps_library_ADCs_adc_16g_asnt_data_a12/1 -> a12/1
  downsample_a13/1 -> delay_a13/1
  xps_library_ADCs_adc_16g_asnt_data_a15/1 -> a15/1
  delay_a12/1 -> xps_library_ADCs_adc_16g_asnt_data_a12/1
  xps_library_ADCs_adc_16g_asnt_data_a14/1 -> a14/1
  downsample_a8/1 -> delay_a8/1
  delay_a10/1 -> xps_library_ADCs_adc_16g_asnt_data_a10/1
  delay_a11/1 -> xps_library_ADCs_adc_16g_asnt_data_a11/1
  delay_a9/1 -> xps_library_ADCs_adc_16g_asnt_data_a9/1
  downsample_a10/1 -> delay_a10/1
  xps_library_ADCs_adc_16g_asnt_data_a9/1 -> a9/1
  downsample_a11/1 -> delay_a11/1
  xps_library_ADCs_adc_16g_asnt_data_a8/1 -> a8/1
  downsample_a9/1 -> delay_a9/1
  xps_library_ADCs_adc_16g_asnt_data_a11/1 -> a11/1
  delay_a8/1 -> xps_library_ADCs_adc_16g_asnt_data_a8/1
  xps_library_ADCs_adc_16g_asnt_data_a10/1 -> a10/1
  downsample_a4/1 -> delay_a4/1
  delay_a6/1 -> xps_library_ADCs_adc_16g_asnt_data_a6/1
  delay_a7/1 -> xps_library_ADCs_adc_16g_asnt_data_a7/1
  delay_a5/1 -> xps_library_ADCs_adc_16g_asnt_data_a5/1
  downsample_a6/1 -> delay_a6/1
  xps_library_ADCs_adc_16g_asnt_data_a5/1 -> a5/1
  downsample_a7/1 -> delay_a7/1
  xps_library_ADCs_adc_16g_asnt_data_a4/1 -> a4/1
  downsample_a5/1 -> delay_a5/1
  xps_library_ADCs_adc_16g_asnt_data_a7/1 -> a7/1
  delay_a4/1 -> xps_library_ADCs_adc_16g_asnt_data_a4/1
  xps_library_ADCs_adc_16g_asnt_data_a6/1 -> a6/1
  sim_a/1 -> gain_a/1
  gain_a/1 -> bias_a/1
  downsample_a0/1 -> delay_a0/1
  delay_a0/1 -> xps_library_ADCs_adc_16g_asnt_data_a0/1
  xps_library_ADCs_adc_16g_asnt_data_a0/1 -> a0/1
  downsample_a1/1 -> delay_a1/1
  delay_a1/1 -> xps_library_ADCs_adc_16g_asnt_data_a1/1
  xps_library_ADCs_adc_16g_asnt_data_a1/1 -> a1/1
  downsample_a2/1 -> delay_a2/1
  delay_a2/1 -> xps_library_ADCs_adc_16g_asnt_data_a2/1
  xps_library_ADCs_adc_16g_asnt_data_a2/1 -> a2/1
  downsample_a3/1 -> delay_a3/1
  delay_a3/1 -> xps_library_ADCs_adc_16g_asnt_data_a3/1
  xps_library_ADCs_adc_16g_asnt_data_a3/1 -> a3/1
  sim_sync/1 -> xps_library_ADCs_adc_16g_asnt_sync/1
